simulink model "TrafficSignalObserver"  (R2024b)
settings: Solver=VariableStepAuto  StartTime=0  StopTime=1000  RelTol=1e-3
PostLoadFcn:
  | helperSLTrafficSignalExampleSetup()
values from neighbouring files (symbols this model uses):
  BusSignalRuntime = Simulink.Bus    [helperSLCreateTrafficSignalBusObjects.m]
  BusSignalSpec = Simulink.Bus    [helperSLCreateTrafficSignalBusObjects.m]
  Ts = 0.02    [HelperReadTrafficSignalRuntime.m]    (also in HelperReadTrafficSignalSpec.m; HelperTrafficSignalFollower.m; TrafficSignalFollowerWithRoadRunnerScenarioExample.m = 0.1; TrafficSignalVisualization.m = 0.05)
undefined symbols (not defined in the file or in its folder): ActorRuntime, Defined, Ego, Lane, m, n, User
libraries: roadrunnerscenario x5
CloseFcn:
  | helperSLTrafficSignalFollowerCleanup
settings Model: Creator=rsuresh  LastModifiedBy=rsuresh
settings SolverCC: DateTimeAtSimulationTimeZero=[]

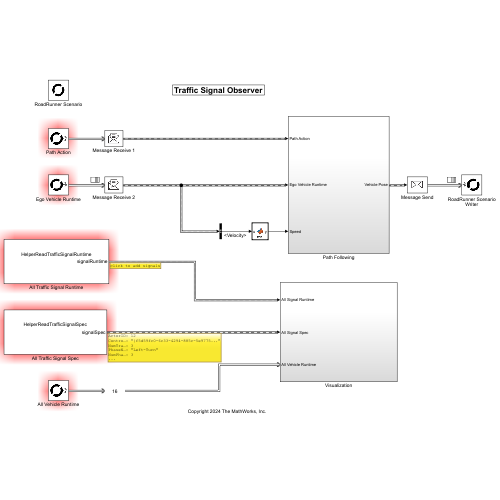
[thumbnail: Simulink's stored preview of the top-level diagram]
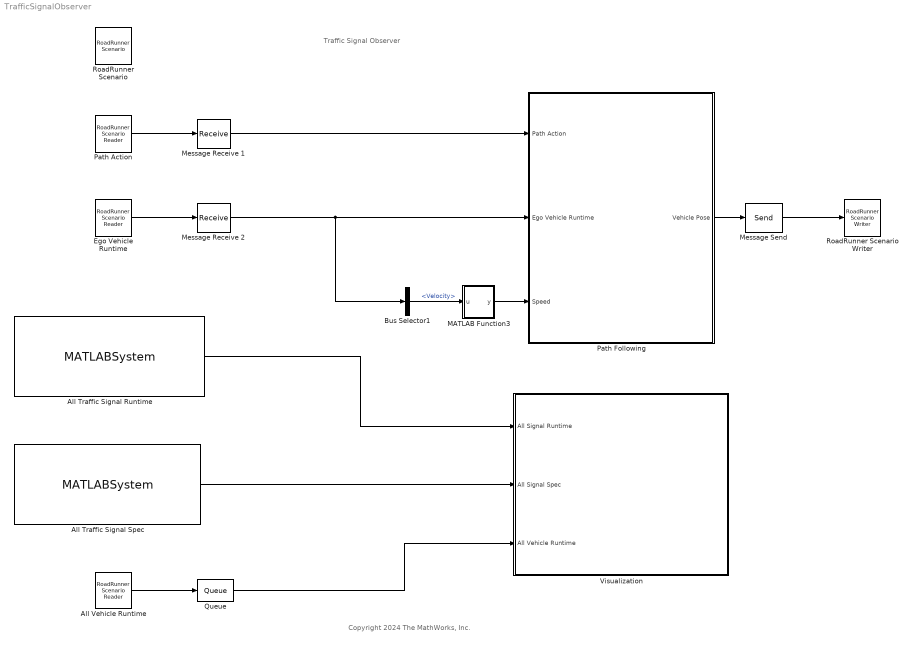
== system TrafficSignalObserver ==
  note: Copyright 2024 The MathWorks, Inc.
  note: Traffic Signal Observer
  All Traffic Signal Runtime : MATLABSystem  System=HelperReadTrafficSignalRuntime  Ts=Ts  OutputStruct="Simulink.Bus.createMATLABStruct(\"BusSignalRuntime\")"
      mask Type: HelperReadTrafficSignalRuntime
      mask Display:
      | disp(['HelperReadTrafficSignalRuntime' char(10) ' ' char(10) ' ' char(10) ' ']);
      | port_label('output',1,'signalRuntime');
  All Traffic Signal Spec : MATLABSystem  System=HelperReadTrafficSignalSpec  Ts=Ts  SignalSpec="Simulink.Bus.createMATLABStruct(\"BusSignalSpec\")"
      mask Type: HelperReadTrafficSignalSpec
      mask Display:
      | disp(['HelperReadTrafficSignalSpec' char(10) ' ' char(10) ' ' char(10) ' ']);
      | port_label('output',1,'signalSpec');
  All Vehicle Runtime : roadrunnerscenario/RoadRunner Scenario Reader  TopicCategory=Actor  ActorCategory=Vehicle  ActionType=Path Following  EventType=User-Defined  TopicType=Actor Pose  VehicleType=Vehicle Pose  UserDefinedAction=Action1  UserDefinedEvent=Event1  Filter=None  SensorTopic=Target Poses  LaneBoundaryOutputTopic=Ego-Lane  SensorID=1  SampleTime=Ts
  Bus Selector1 : BusSelector  OutputSignals=ActorRuntime.Velocity
  Ego Vehicle Runtime : roadrunnerscenario/RoadRunner Scenario Reader  TopicCategory=Actor  ActorCategory=Vehicle  ActionType=Path Following  EventType=User-Defined  TopicType=Actor Pose  VehicleType=Vehicle Pose  UserDefinedAction=Action1  UserDefinedEvent=Event1  Filter=Self  SensorTopic=Target Poses  LaneBoundaryOutputTopic=Ego-Lane  SensorID=1  SampleTime=Ts
  MATLAB Function3 : MATLAB Function  TreatAsAtomicUnit=on
  Message Receive 1 : Receive  InputPortMessageModes=m
  Message Receive 2 : Receive  InputPortMessageModes=m  UseInternalQueue=off  QueueOverwriting=on  QueueLength=1  QueueType=LIFO
  Message Send : Send  OutputPortMessageModes=m
  Path Action : roadrunnerscenario/RoadRunner Scenario Reader  TopicCategory=Action  ActorCategory=All Types  ActionType=Path Following  EventType=User-Defined  TopicType=Actor Specifications  VehicleType=Vehicle Specifications  UserDefinedAction=Action1  UserDefinedEvent=Event1  Filter=Self  SensorTopic=Target Poses  LaneBoundaryOutputTopic=Ego-Lane  SensorID=1  SampleTime=Ts
  Path Following : Subsystem
  Queue : Queue  InputPortMessageModes=m  OutputPortMessageModes=m  OverwriteOldest=on  Capacity=16
  RoadRunner Scenario : roadrunnerscenario/RoadRunner Scenario  UserDefinedActions={}  UserDefinedEvents={}
  RoadRunner Scenario Writer : roadrunnerscenario/RoadRunner Scenario Writer  TopicCategory=Actor  ActorCategory=Vehicle  EventType=Action Complete  UserDefinedEvent=Event1  VehicleType=Vehicle Pose  TopicType=Actor Pose
  Visualization : Subsystem
  wires:
  Path Following/1(Vehicle Pose) -> Message Send/1
  Message Send/1 -> RoadRunner Scenario Writer/1
  Ego Vehicle Runtime/1 -> Message Receive 2/1
  Message Receive 2/1 -> Path Following/2(Ego Vehicle Runtime), Bus Selector1/1
  Path Action/1 -> Message Receive 1/1
  All Vehicle Runtime/1 -> Queue/1
  Queue/1 -> Visualization/3(All Vehicle Runtime)
  MATLAB Function3/1(y) -> Path Following/3(Speed)
  Message Receive 1/1 -> Path Following/1(Path Action)
  Bus Selector1/1 -> MATLAB Function3/1(u)  "<Velocity>"
  All Traffic Signal Spec/1 -> Visualization/2(All Signal Spec)
  All Traffic Signal Runtime/1 -> Visualization/1(All Signal Runtime)

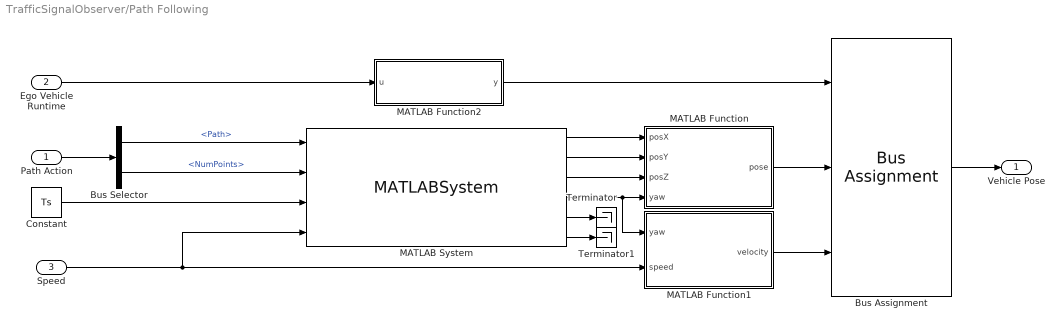
== system TrafficSignalObserver/Path Following ==
  Path Action : Inport
  Ego Vehicle Runtime : Inport  Port=2
  Speed : Inport  Port=3
  Bus Assignment : BusAssignment  AssignedSignals=ActorRuntime.Pose,ActorRuntime.Velocity
  Bus Selector : BusSelector  OutputSignals=PathTarget.Path,PathTarget.NumPoints
  Constant : Constant  Value=Ts
  MATLAB Function : MATLAB Function  TreatAsAtomicUnit=on
  MATLAB Function1 : MATLAB Function  TreatAsAtomicUnit=on
  MATLAB Function2 : MATLAB Function  TreatAsAtomicUnit=on
  MATLAB System : MATLABSystem  System=HelperPolylineEvaluator  SimulateUsing=Code generation
      mask Type: HelperPolylineEvaluator
      mask Display:
      | disp('HelperPolylineEvaluator');
      | port_label('input',1,'polyline');
      | port_label('input',2,'polylineLength');
      | port_label('input',3,'timestep');
      | port_label('input',4,'speed');
      | port_label('output',1,'posX');
      | port_label('output',2,'posY');
      | port_label('output',3,'posZ');
      | port_label('output',4,'yaw');
      | port_label('output',5,'routeDistance');
      | port_label('output',6,'routeFinished');
  Terminator : Terminator
  Terminator1 : Terminator
  Vehicle Pose : Outport
  wires:
  Constant/1 -> MATLAB System/3
  MATLAB System/2 -> MATLAB Function/2(posY)
  MATLAB System/1 -> MATLAB Function/1(posX)
  MATLAB Function2/1(y) -> Bus Assignment/1
  Bus Selector/1 -> MATLAB System/1  "<Path>"
  MATLAB System/5 -> Terminator/1
  MATLAB System/6 -> Terminator1/1
  MATLAB Function1/1(velocity) -> Bus Assignment/3
  MATLAB Function/1(pose) -> Bus Assignment/2
  Bus Selector/2 -> MATLAB System/2  "<NumPoints>"
  MATLAB System/3 -> MATLAB Function/3(posZ)
  Ego Vehicle Runtime/1 -> MATLAB Function2/1(u)
  Path Action/1 -> Bus Selector/1
  Bus Assignment/1 -> Vehicle Pose/1
  MATLAB System/4 -> MATLAB Function/4(yaw), MATLAB Function1/1(yaw)
  Speed/1 -> MATLAB Function1/2(speed), MATLAB System/4

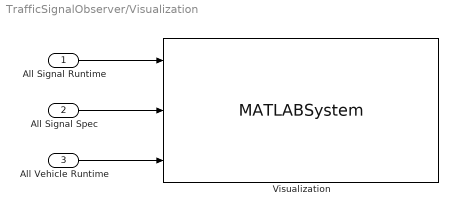
== system TrafficSignalObserver/Visualization ==
  All Signal Runtime : Inport
  All Signal Spec : Inport  Port=2
  All Vehicle Runtime : Inport  Port=3
  Visualization : MATLABSystem  InputPortMessageModes=n,n,m  System=TrafficSignalVisualization  RRHDMap=rrHDMap  VehicleSpec=vehicleSpec  EgoControllerID=controllerID  EgoSignalID=signalID  EgoID=egoActorID  Ts=Ts  DisableVisualization=off
      mask Type: TrafficSignalVisualization
      mask Display:
      | disp(['TrafficSignalVisualization' char(10) ' ' char(10) ' ' char(10) ' ']);
      | port_label('input',1,'signalRuntime');
      | port_label('input',2,'signalSpec');
      | port_label('input',3,'allVehicleRuntime');
  wires:
  All Signal Runtime/1 -> Visualization/1
  All Signal Spec/1 -> Visualization/2
  All Vehicle Runtime/1 -> Visualization/3

== matlab function TrafficSignalObserver/Path Following/MATLAB Function1 ==
  data: yaw input; speed input; velocity output
function velocity = getVehVel(yaw,speed)
    velocity = speed*[-sin(yaw) cos(yaw) 0];
end

== matlab function TrafficSignalObserver/Path Following/MATLAB Function ==
  data: posX input; pose output; posY input; posZ input; yaw input
function pose = packActorPose(posX, posY, posZ, yaw)
    % Pack the pose into 4x4 matrix.
    Position = [posX posY posZ];
    Rotation = [yaw 0 0];
    % Get rotation matrix
    rotm = eul2rotm(Rotation);            
    pose = [[rotm Position']; [0 0 0 1]];
end

== matlab function TrafficSignalObserver/Path Following/MATLAB Function2 ==
  data: u input Bus: BusVehicleRuntime; y output Bus: BusVehicleRuntime
function y = fcn(u)

y = u;

== matlab function TrafficSignalObserver/MATLAB Function3 ==
  data: u input; y output
function y = fcn(u)

y = norm(u);
